simulink model "LQG_NL_Final"  (R2019b)
settings: Solver=VariableStepAuto  StartTime=0.0  StopTime=200  RelTol=1e-3
undefined symbols (not defined in the file): A, B, C, Continuous, D, K, Time
libraries: ctrlSharedLib x1
settings Model: Creator=Pranali  LastModifiedBy=shubh
settings DataIOCC: ReturnWorkspaceOutputs=off
settings DebuggingCC: ArithmeticOperatorsInVariantConditions=warning
settings SFSimCC: CustomCodeUndefinedFunction=UseInterfaceOnly

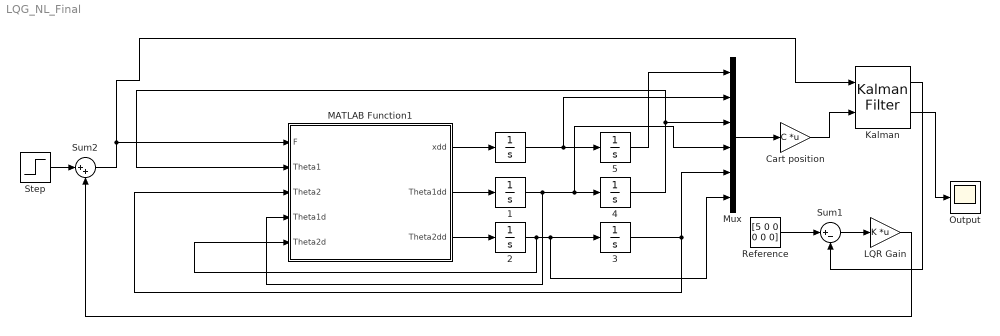
== system LQG_NL_Final ==
   {,1..5} (6 alike) : Integrator
  Cart position : Gain  Gain=C  Multiplication=Matrix(K*u)
  Kalman : ctrlSharedLib/Kalman Filter  TimeDomain=Continuous-Time  UseCurrentEstimator=on  ModelSource=Individual A, B, C, D matrices  ModelSourceVariable=ss(A,B,C,D)  A=A  B=B  C=C  D=0  NumberOfStates=1  NumberOfInputs=1  NumberOfOutputs=1  InitialEstimateSource=Dialog  X0=[1 0 pi/12 0 pi/12 0]  P0=10  UseK=off  UseGH=off  NumberOfProcessNoiseInputs=1  G=1  TimeInvariantG=on  H=0  TimeInvariantH=on  Q=1  TimeInvariantQ=on  R=1  TimeInvariantR=on  N=0  TimeInvariantN=on  AddInputPort=on  AddEnablePort=off  OutputEstimatedY=on  OutputP=off  Ts=-1
      settings: SourceProductBaseCode=CT
  LQR Gain : Gain  Gain=K  Multiplication=Matrix(K*u)
  MATLAB Function1 : MATLAB Function  TreatAsAtomicUnit=on
  Mux : Mux  Inputs=6
  Output : Scope
  "Reference " : Constant  Value=[5 0 0 0 0 0]
  Step : Step  Time=10  SampleTime=0
  Sum1 : Sum  Inputs=|+-
  Sum2 : Sum  Inputs=|++
  wires:
  MATLAB Function1/2(Theta1dd) -> " 1"/1
  Mux/1 -> Cart position/1
  Step/1 -> Sum2/1
  " 4"/1 -> MATLAB Function1/2(Theta1), Mux/3
  " "/1 -> " 5"/1, Mux/2
  " 3"/1 -> MATLAB Function1/3(Theta2), Mux/5
  Cart position/1 -> Kalman/2
  " 1"/1 -> MATLAB Function1/4(Theta1d), " 4"/1, Mux/4
  MATLAB Function1/3(Theta2dd) -> " 2"/1
  MATLAB Function1/1(xdd) -> " "/1
  " 2"/1 -> MATLAB Function1/5(Theta2d), " 3"/1, Mux/6
  " 5"/1 -> Mux/1
  Kalman/2 -> Output/1
  Kalman/1 -> Sum1/2
  "Reference "/1 -> Sum1/1
  LQR Gain/1 -> Sum2/2
  Sum1/1 -> LQR Gain/1
  Sum2/1 -> MATLAB Function1/1(F), Kalman/1

== matlab function LQG_NL_Final/MATLAB Function1 ==
  data: F input; Theta1 input; Theta2 input; xdd output; Theta1d input; Theta2d input; Theta1dd output; Theta2dd output
function [xdd,Theta1dd,Theta2dd] = NL_LQG(F,Theta1,Theta2,Theta1d,Theta2d)
l1 = 20; 
l2 = 10; 
m1 = 100; 
m2 = 100; 
M = 1000; 
g = 9.81; 
xdd = (F - m1*cos(Theta1)*sin(Theta1)*g - m2*cos(Theta2)*sin(Theta2)*g - m1*l1*(Theta1d^2)*(sin(Theta1)) - m2*l2*(Theta2d^2)*(sin(Theta2)))/(M + m1*(sin(Theta1)^2) + m2*(sin(Theta2)^2));
Theta1dd = (xdd*cos(Theta1) - g*sin(Theta1))/l1;
Theta2dd = (xdd*cos(Theta2) - g*sin(Theta2))/l2;
end
